simulink model "flight_dynamics_3"  (R2016b)
settings: Solver=FixedStepAuto  StartTime=0.0  StopTime=inf  FixedStep=.0005  RelTol=1e-3  EnableMultiTasking=on
InitFcn:
  | param
undefined symbols (not defined in the file or in its folder): drawAircraft
libraries: simulink x6
settings Model: Creator=nmd89  LastModifiedBy=nmd89
settings OptimizationCC: LifeSpan=inf
settings DebuggingCC: SFUnexpectedBacktrackingDiag=warning  SFNoUnconditionalDefaultTransitionDiag=warning  SFExecutionAtInitializationDiag=none
settings GRTTargetCC: TargetLangStandard=C89/C90 (ANSI)  GeneratePreprocessorConditionals=Disable all
settings ConfigComp: CovMetricSettings=dw  CovHtmlReporting=on  CovSaveCumulativeToWorkspaceVar=on  CovSaveSingleToWorkspaceVar=on  CovExternalEMLEnable=off

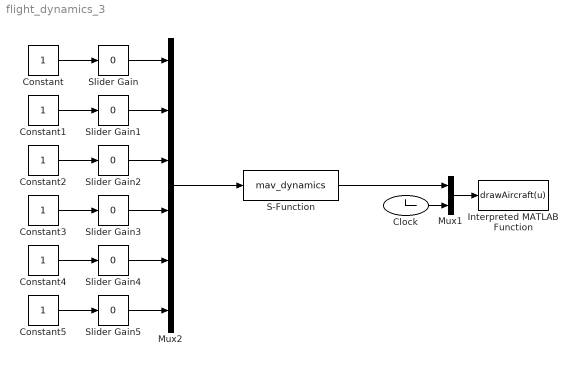
== system flight_dynamics_3 ==
  Clock : Clock
  Constant{,1..5} (6 alike) : Constant
  Interpreted MATLAB Function : MATLABFcn  MATLABFcn=drawAircraft(u)  OutputDimensions=0
  Mux1 : Mux  Inputs=2
  Mux2 : Mux  Inputs=6
  S-Function : S-Function  FunctionName=mav_dynamics  Parameters=P  SFunctionDeploymentMode=off  EnableBusSupport=off
  Slider Gain{,1..5} (6 alike) : simulink/Math Operations/Slider Gain  low=-40  gain=0  high=40
  wires:
  Mux1/1 -> Interpreted MATLAB Function/1
  Clock/1 -> Mux1/2
  S-Function/1 -> Mux1/1
  Slider Gain/1 -> Mux2/1
  Constant/1 -> Slider Gain/1
  Constant1/1 -> Slider Gain1/1
  Constant2/1 -> Slider Gain2/1
  Slider Gain2/1 -> Mux2/3
  Constant3/1 -> Slider Gain3/1
  Slider Gain3/1 -> Mux2/4
  Constant4/1 -> Slider Gain4/1
  Slider Gain4/1 -> Mux2/5
  Constant5/1 -> Slider Gain5/1
  Slider Gain5/1 -> Mux2/6
  Slider Gain1/1 -> Mux2/2
  Mux2/1 -> S-Function/1
